simulink model "force_optimize"  (R2013a)
settings: Solver=FixedStepDiscrete  StartTime=0.0  StopTime=80  FixedStep=.001  RelTol=1e-3
libraries: simulink x3
settings Model: Creator=dholley  LastModifiedBy=dholley
settings DataIOCC: LimitDataPoints=off

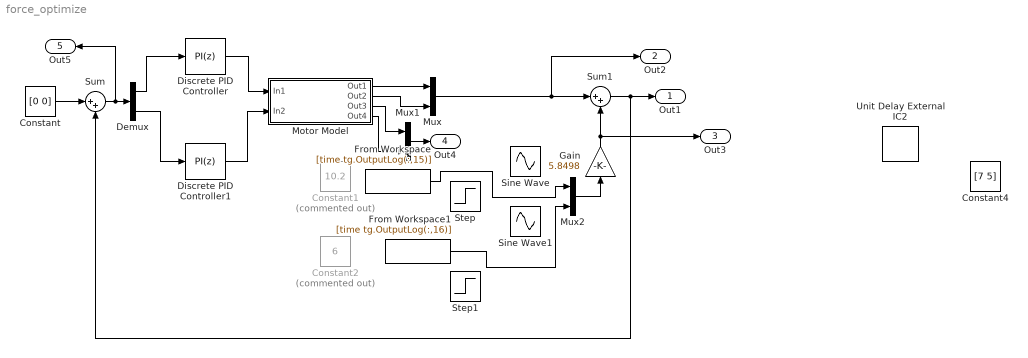
== system force_optimize ==
  Constant : Constant  Value=[0 0]
  Constant1 : Constant  Commented=on  Value=10.2
  Constant2 : Constant  Commented=on  Value=6
  Constant4 : Constant  Value=[7 5]
  Demux : Demux  Outputs=2
  Discrete PID Controller : simulink/Continuous/PID Controller  Controller=PI  TimeDomain=Discrete-time  SampleTime=.001  IntegratorMethod=Forward Euler  FilterMethod=Forward Euler  Form=Parallel  P=.01  I=100  D=0  N=100  InitialConditionSource=internal  InitialConditionForIntegrator=0  InitialConditionForFilter=0  ExternalReset=none  LimitOutput=off  UpperSaturationLimit=inf  LowerSaturationLimit=-inf  LinearizeAsGain=off  AntiWindupMode=none  Kb=1  TrackingMode=off  Kt=1  PParamMin=[]  PParamMax=[]  IParamMin=[]  IParamMax=[]  DParamMin=[]  DParamMax=[]  NParamMin=[]  NParamMax=[]  KbParamMin=[]  KbParamMax=[]  KtParamMin=[]  KtParamMax=[]  POutMin=[]  POutMax=[]  IOutMin=[]  IOutMax=[]  DOutMin=[]  DOutMax=[]  NOutMin=[]  NOutMax=[]  KbOutMin=[]  KbOutMax=[]  KtOutMin=[]  KtOutMax=[]  IntegratorOutMin=[]  IntegratorOutMax=[]  FilterOutMin=[]  FilterOutMax=[]  SumOutMin=[]  SumOutMax=[]  SumI1OutMin=[]  SumI1OutMax=[]  SumI2OutMin=[]  SumI2OutMax=[]  SumI3OutMin=[]  SumI3OutMax=[]  SumDOutMin=[]  SumDOutMax=[]  SaturationOutMin=[]  SaturationOutMax=[]  IntegratorContinuousStateAttributes=''  IntegratorStateMustResolveToSignalObject=off  IntegratorRTWStateStorageClass=Auto  FilterContinuousStateAttributes=''  FilterStateMustResolveToSignalObject=off  FilterRTWStateStorageClass=Auto
  Discrete PID Controller1 : simulink/Continuous/PID Controller  Controller=PI  TimeDomain=Discrete-time  SampleTime=.001  IntegratorMethod=Forward Euler  FilterMethod=Forward Euler  Form=Parallel  P=.01  I=100  D=0  N=100  InitialConditionSource=internal  InitialConditionForIntegrator=0  InitialConditionForFilter=0  ExternalReset=none  LimitOutput=off  UpperSaturationLimit=inf  LowerSaturationLimit=-inf  LinearizeAsGain=off  AntiWindupMode=none  Kb=1  TrackingMode=off  Kt=1  PParamMin=[]  PParamMax=[]  IParamMin=[]  IParamMax=[]  DParamMin=[]  DParamMax=[]  NParamMin=[]  NParamMax=[]  KbParamMin=[]  KbParamMax=[]  KtParamMin=[]  KtParamMax=[]  POutMin=[]  POutMax=[]  IOutMin=[]  IOutMax=[]  DOutMin=[]  DOutMax=[]  NOutMin=[]  NOutMax=[]  KbOutMin=[]  KbOutMax=[]  KtOutMin=[]  KtOutMax=[]  IntegratorOutMin=[]  IntegratorOutMax=[]  FilterOutMin=[]  FilterOutMax=[]  SumOutMin=[]  SumOutMax=[]  SumI1OutMin=[]  SumI1OutMax=[]  SumI2OutMin=[]  SumI2OutMax=[]  SumI3OutMin=[]  SumI3OutMax=[]  SumDOutMin=[]  SumDOutMax=[]  SaturationOutMin=[]  SaturationOutMax=[]  IntegratorContinuousStateAttributes=''  IntegratorStateMustResolveToSignalObject=off  IntegratorRTWStateStorageClass=Auto  FilterContinuousStateAttributes=''  FilterStateMustResolveToSignalObject=off  FilterRTWStateStorageClass=Auto
  From Workspace : FromWorkspace  VariableName=[time tg.OutputLog(:,15)]  SampleTime=0
  From Workspace1 : FromWorkspace  VariableName=[time tg.OutputLog(:,16)]  SampleTime=0
  Gain : Gain  Gain=5.8498
  Motor Model : Subsystem
  Mux : Mux  Inputs=2
  Mux1 : Mux  Inputs=2
  Mux2 : Mux  Inputs=2
  Sine Wave : Sin  Amplitude=5  Frequency=3.1416  SampleTime=0
  Sine Wave1 : Sin  Amplitude=-5  Frequency=3.1416  SampleTime=0
  Step : Step  After=5  SampleTime=0
  Step1 : Step  After=3  SampleTime=0
  Sum : Sum  Inputs=|++
  Sum1 : Sum  Inputs=|++
  Unit Delay External IC2 : simulink/Additional Math & Discrete/Additional Discrete/Unit Delay External IC  tsamp=.001
  Out1 : Outport
  Out2 : Outport  Port=2
  Out3 : Outport  Port=3
  Out4 : Outport  Port=4
  Out5 : Outport  Port=5
  wires:
  Sum/1 -> Out5/1, Demux/1
  Motor Model/1(Out1) -> Mux/1
  Sum1/1 -> Sum/2, Out1/1
  Constant/1 -> Sum/1
  Motor Model/2(Out2) -> Mux/2
  Mux1/1 -> Out4/1
  Motor Model/3(Out3) -> Mux1/1
  Motor Model/4(Out4) -> Mux1/2
  Mux/1 -> Out2/1, Sum1/1
  Mux2/1 -> Gain/1
  Demux/1 -> Discrete PID Controller/1
  Demux/2 -> Discrete PID Controller1/1
  Discrete PID Controller1/1 -> Motor Model/2(In2)
  Discrete PID Controller/1 -> Motor Model/1(In1)
  From Workspace/1 -> Mux2/1
  From Workspace1/1 -> Mux2/2
  Gain/1 -> Out3/1, Sum1/2

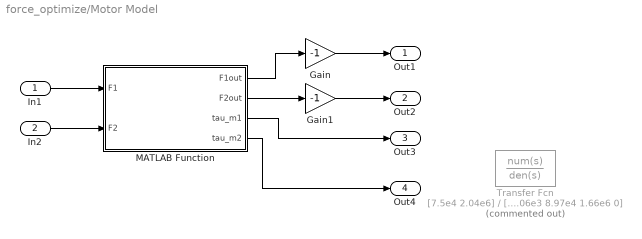
== system force_optimize/Motor Model ==
  In1 : Inport
  In2 : Inport  Port=2
  Gain : Gain  Gain=-1
  Gain1 : Gain  Gain=-1
  MATLAB Function : MATLAB Function  TreatAsAtomicUnit=on
  Transfer Fcn : TransferFcn  Commented=on  Numerator=[7.5e4 2.04e6]  Denominator=[.0898 1.06e3 8.97e4 1.66e6 0]
  Out1 : Outport
  Out2 : Outport  Port=2
  Out3 : Outport  Port=3
  Out4 : Outport  Port=4
  wires:
  MATLAB Function/1(F1out) -> Gain/1
  In1/1 -> MATLAB Function/1(F1)
  In2/1 -> MATLAB Function/2(F2)
  MATLAB Function/2(F2out) -> Gain1/1
  Gain/1 -> Out1/1
  Gain1/1 -> Out2/1
  MATLAB Function/3(tau_m1) -> Out3/1
  MATLAB Function/4(tau_m2) -> Out4/1

== matlab function force_optimize/Motor Model/MATLAB Function ==
  data: F1 input; F1out output; F2 input; F2out output; tau_m1 output; tau_m2 output
function [F1out,F2out,tau_m1,tau_m2] = f2t(F1,F2)
%#codegen


%Revision 8/12/14
F1ps=(F1/2.7)-(F2/1.588);
F1fe=(F1+F2)/1.588;
F2ps=(-F1/2.7)+(F2/1.588);
F2fe=(F1+F2)/2.7;


Ffe=((10*F1fe)+(17*F2fe))/27;
Fps=(F1ps-F2ps)/2;

tau_m1=Fps/.4956;
tau_m2=Ffe/1.26643;

F1out=(.5884*tau_m1)+(.5049*tau_m2);
F2out=(-.3472*tau_m1)+(1.5928*tau_m2);


end
